simulink model "sl_subsys_for2"  (Simulink 6.0)
settings: Solver=FixedStepDiscrete  StartTime=0.0  StopTime=10.0  FixedStep=1  RelTol=1e-3
settings Model: Creator=The MathWorks Inc.  LastModifiedBy=batserve  ExtModeAutoUpdateStatusClock=off
settings OptimizationCC: BooleanDataType=off
settings DebuggingCC: CheckExecutionContextPreStartOutputMsg=on  CheckExecutionContextRuntimeOutputMsg=on  SolverPrmCheckMsg=none
settings HardwareCC: TargetUnknown=on

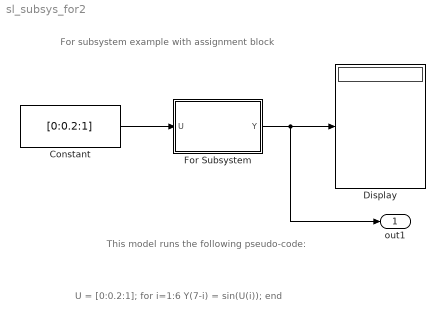
== system sl_subsys_for2 ==
  note: This model runs the following pseudo-code:
  note: U = [0:0.2:1];
      |       for i=1:6
      |                            Y(7-i) = sin(U(i));
      | end
  note: For subsystem example with assignment block
  Constant : Constant  Value=[0:0.2:1]
  Display : Display
  For Subsystem : Subsystem  TreatAsAtomicUnit=on  PropExecContextAcrossSSBoundary=on
  out1 : Outport
  wires:
  Constant/1 -> For Subsystem/1(U)
  For Subsystem/1(Y) -> Display/1, out1/1

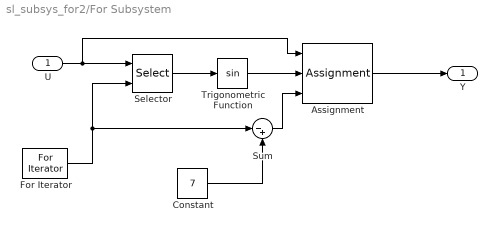
== system sl_subsys_for2/For Subsystem ==
  U : Inport  Port=1  LatchInput=off
  Assignment : Assignment  ElementSrc=External
  Constant : Constant  Value=7
  For Iterator : ForIterator  ResetStates=reset  IterationLimit=6  IterationVariableDataType=double
  Selector : Selector  ElementSrc=External  Elements=[1 3]
  Sum : Sum  Inputs=|-+  SaturateOnIntegerOverflow=on  InputSameDT=on
  Trigonometric Function : Trigonometry
  Y : Outport
  wires:
  For Iterator/1 -> Selector/2, Sum/1
  U/1 -> Selector/1, Assignment/1
  Selector/1 -> Trigonometric Function/1
  Assignment/1 -> Y/1
  Trigonometric Function/1 -> Assignment/2
  Constant/1 -> Sum/2
  Sum/1 -> Assignment/3
